simulink model "queuetest_fifth"  (R2018a)
settings: Solver=VariableStepAuto  StartTime=0.0  StopTime=20.0  RelTol=1e-3
undefined symbols (not defined in the file or in its folder): m, n
settings Model: Creator=Michael Girbino  LastModifiedBy=Michael Girbino
settings DebuggingCC: SFNoUnconditionalDefaultTransitionDiag=warning  SFOutputUsedAsStateInMooreChartDiag=warning

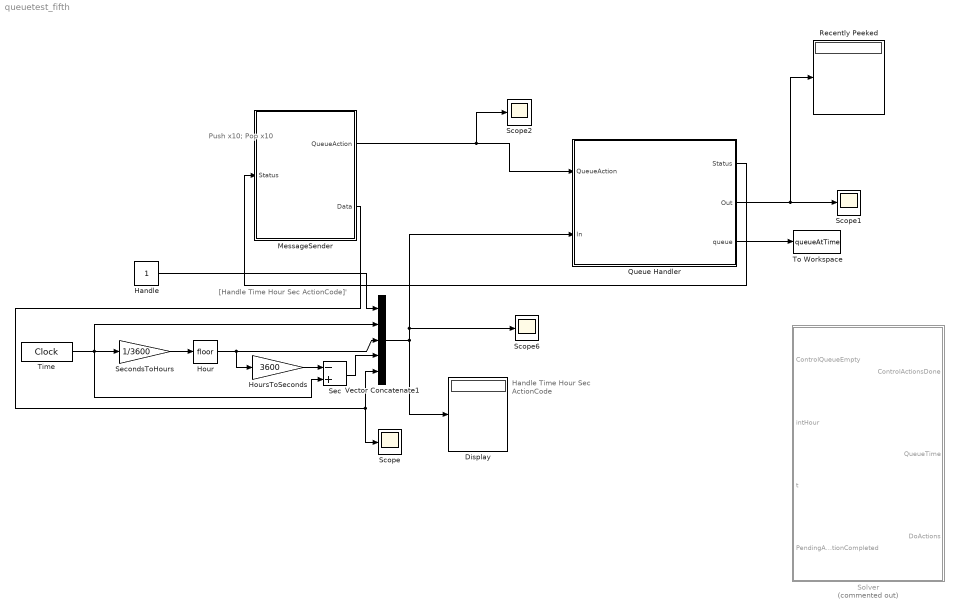
== system queuetest_fifth ==
  note: Push x10;
      | Pop x10
  note: [Handle Time Hour Sec ActionCode]'
  note: Handle
      | Time
      | Hour
      | Sec
      | ActionCode
  Display : Display
  Handle : Constant
  Hour : Rounding
  HoursToSeconds : Gain  Gain=3600
  MessageSender : Stateflow chart  TreatAsAtomicUnit=on
  Queue Handler : Stateflow chart  TreatAsAtomicUnit=on
  Recently Peeked : Display
  Scope{,1..2,6} (4 alike) : Scope
  Sec : Sum  Inputs=-+
  SecondsToHours : Gain  Gain=1/3600
  Solver : Stateflow chart  Commented=on  TreatAsAtomicUnit=on
  Time : DigitalClock
  To Workspace : ToWorkspace  VariableName=queueAtTime  SaveFormat=Structure With Time  SampleTime=-1
  Vector Concatenate1 : Concatenate  NumInputs=5
  wires:
  MessageSender/1(QueueAction) -> Scope2/1, Queue Handler/1(QueueAction)
  MessageSender/2(Data) -> Scope/1, Vector Concatenate1/5
  Queue Handler/1(Status) -> MessageSender/1(Status)
  Queue Handler/2(Out) -> Scope1/1, Recently Peeked/1
  Hour/1 -> Vector Concatenate1/3, HoursToSeconds/1
  Time/1 -> Vector Concatenate1/2, Sec/2, SecondsToHours/1
  SecondsToHours/1 -> Hour/1
  HoursToSeconds/1 -> Sec/1
  Sec/1 -> Vector Concatenate1/4
  Queue Handler/3(queue) -> To Workspace/1
  Handle/1 -> Vector Concatenate1/1
  Vector Concatenate1/1 -> Scope6/1, Queue Handler/2(In), Display/1

== stateflow chart queuetest_fifth/Solver ==
  (default) -> (junction 25) : % Execute control actions in order based on control mode
  (junction 25) -> (junction 26) [order 1] : [ControlMode == ControlModes.STATIC]
  (junction 25) -> (junction 29) [order 2]
  (junction 26) -> (junction 54)
  (junction 54) -> (junction 55) [order 1] : [ControlQueueEmpty]
      | % execute nearest set of control actions, but leave time where it is
  (junction 54) -> (junction 56) [order 2] : {QueueTime = [0,0]; %xHour, xSec
      | DoActions.data = QueueOps.NearestActions;
      | send(DoActions);
      | % ignores time advancement
      | }
  (junction 55) -> (junction 57) : {ControlActionsDone = true;}
  (junction 57) -> (junction 56)
  (junction 56) -> (junction 27)
  (junction 27) -> (junction 28)
  (junction 28) -> (junction 32)
  (junction 29) -> (junction 30) [order 1] : [ControlMode == ControlModes.EVENTDRIVEN]
      | % execute nearest set of control actions and advance time to that time
  (junction 30) -> (junction 65) : {QueueTime = [intHour,t]; %xHour, xSec
      | DoActions.data = QueueOps.NearestActions;
      | send(DoActions);}
  (junction 29) -> (junction 33) [order 2]
  (junction 65) -> (junction 66) [order 1] : [~PendingActionCompleted]
  (junction 65) -> (junction 67) [order 2]
  (junction 66) -> (junction 68) : {ControlActionsDone = true;
      | % advances time to the next event
      | }
  (junction 68) -> (junction 67)
  (junction 67) -> (junction 31)
  (junction 31) -> (junction 32)
  (junction 32) -> (junction 36)
  (junction 33) -> (junction 34) [order 1] : [ControlMode == ControlModes.TIMEDRIVEN]
      |  % Do all actions having and action time <= specified time
  (junction 33) -> (junction 37) [order 2]
  (junction 34) -> (junction 78) : {QueueTime = [intHour,t]; %xHour, xSec
      | DoActions.data = QueueOps.JustActions;
      | send(DoActions);}
  (junction 78) -> (junction 80) [order 1] : [~PendingActionCompleted]
  (junction 78) -> (junction 79) [order 2]
  (junction 80) -> (junction 82) : {ControlActionsDone = true;
      | }
  (junction 82) -> (junction 79)
  (junction 79) -> (junction 35)
  (junction 35) -> (junction 36)
  (junction 36) -> (junction 40)
  (junction 37) -> (junction 38) [order 1] : [ControlMode == ControlModes.MULTIRATE]
      |  % Execute the nearest set of control actions, but leave time where it is
  (junction 37) -> (junction 41) [order 2]
  (junction 38) -> (junction 91) : {QueueTime = [intHour,t]; %xHour, xSec
      | DoActions.data = QueueOps.MultiRate;
      | send(DoActions);}
  (junction 91) -> (junction 88) [order 1] : [~PendingActionCompleted]
  (junction 91) -> (junction 87) [order 2]
  (junction 88) -> (junction 92) : {ControlActionsDone = true;
      | }
  (junction 92) -> (junction 87)
  (junction 87) -> (junction 39)
  (junction 39) -> (junction 40)
  (junction 40) -> (junction 42)
  (junction 42) -> (junction 41)
  (junction 41) -> (junction 43)
  data: ControlQueueEmpty input boolean; ControlActionsDone output boolean; QueueTime output double size=2; DoActions output double; intHour input uint8; t input uint32; PendingActionCompleted input boolean

== stateflow chart queuetest_fifth/MessageSender ==
  settings: enableNonTerminalStates=1
  state SayPush
    en:
    Data = ii;
    QueueAction.data = ...
    QueueActions.PUSH;
    send(QueueAction);
    ii = ii+1;
  state SayPeek
    en:
    QueueAction.data = ...
    QueueActions.PEEK;
    send(QueueAction);
  state SayDoAllACtions
    en:
    QueueAction.data = ...
    QueueActions.DO_ALL_ACTIONS;
    send(QueueAction);
  state SayPop [commented out]
    en:
    QueueAction.data = ...
    QueueActions.POP;
    send(QueueAction);
    ii = ii+1;
  state Asleep
  (default) -> SayPush : {ii = 1;}
  (junction 21) -> SayPush [order 1] : [ii <= 10]
  SayPush -> Asleep [order 2] : Status[Status.data == Statuses.ERROR]
  SayPush -> (junction 21) [order 1] : Status[Status.data == Statuses.READY]
  (junction 21) -> SayPeek [order 2]
  SayPeek -> Asleep [order 2] : Status[Status.data==Statuses.ERROR]
  SayPeek -> (junction 51) [order 1] : Status[Status.data == Statuses.READY]
  (junction 51) -> SayDoAllACtions
  SayDoAllACtions -> Asleep [order 1] : Status[Status.data==Statuses.ERROR]
  SayDoAllACtions -> Asleep [order 2] : {ii = 1;
      | Data = 0;}
  (junction 25) -> SayPop [commented out] : [ii <= 10]
  SayPop -> Asleep [commented out] : Status[Status.data == Statuses.ERROR]
  SayPop -> (junction 25) [commented out] : Status[Status.data == Statuses.READY]
  (junction 25) -> Asleep [commented out]
  data: QueueAction output Enum: QueueActions; Data output double size=1; Status input Enum: Statuses; ii local double =0

== stateflow chart queuetest_fifth/Queue Handler ==
  settings: enableNonTerminalStates=1
  state Executive [parallel]
    settings: executionOrder=1
    state Asleep
      ex: Status.data = Statuses.READY; % reset status
      INTERNAL_DONE = false;
      EXECUTIVE_DONE = false;
    state DoNearestActions
      state WaitOnPeek
        en: send(QUEUE_PEEK, Internal);
      state WaitOnPop
        en: send(QUEUE_POP, Internal);
      state ErrorNoItems
        en: Status.data = ...
        Statuses.ERROR;
        send(Status);
      (default) -> (junction 302) : % do only those actions with the same delay time as the first action time return time
          | {q_len_initial = GetQueueSize;
          | PendingActionsCompleted = false; % local for now
          | }
      (junction 302) -> (junction 315) [order 1] : [q_len_initial > 0]
      (junction 302) -> Executive.DoNearestActions.ErrorNoItems [order 2]
      (junction 315) -> Executive.DoNearestActions.WaitOnPeek : {INTERNAL_DONE = false;}
      (junction 301) -> (junction 331) [order 1] : [jj <= q_len_initial]
      (junction 331) -> Executive.DoNearestActions.WaitOnPop : {INTERNAL_DONE = false;}
      Executive.DoNearestActions.WaitOnPeek -> (junction 301) : [INTERNAL_DONE]
          | {ActionTime = Out(QF.Time);
          | QHour = Out(QF.Hour);
          | QSec = Out(QF.Sec);
          | jj = 1;}
      Executive.DoNearestActions.WaitOnPop -> (junction 299) : [INTERNAL_DONE]
          | %send(DoPendingAction);
      (junction 299) -> (junction 301) : {jj = jj + 1;}
      (junction 301) -> (junction 305) [order 2]
      Executive.DoNearestActions.ErrorNoItems -> (junction 300)
      (junction 305) -> (junction 300)
      (junction 300) -> (junction 298) : {EXECUTIVE_DONE = true;}
    state DoAllActions
      state WaitOnPop
        en: send(QUEUE_POP, Internal);
      state ErrorNoItems
        en: Status.data = ...
        Statuses.ERROR;
        send(Status);
      (default) -> (junction 322) : {q_len_initial = GetQueueSize;}
      (junction 322) -> (junction 321) [order 1] : [q_len_initial ~= 0]
      (junction 322) -> Executive.DoAllActions.ErrorNoItems [order 2]
      (junction 321) -> (junction 326) : {jj = 1;}
      (junction 326) -> (junction 316) [order 1] : [jj <= q_len_initial]
      (junction 316) -> Executive.DoAllActions.WaitOnPop : {INTERNAL_DONE = false;}
      (junction 314) -> (junction 326) : {jj = jj + 1;}
      (junction 326) -> (junction 312) [order 2]
      Executive.DoAllActions.WaitOnPop -> (junction 314) : [INTERNAL_DONE]
          | %send(DoPendingAction);
      Executive.DoAllActions.ErrorNoItems -> (junction 324)
      (junction 312) -> (junction 324)
      (junction 324) -> (junction 310) : {EXECUTIVE_DONE = true;}
    state Pushing
      en: send(QUEUE_PUSH, Internal);
    state Peeking
      en: send(QUEUE_PEEK, Internal);
    state Popping
      en: send(QUEUE_POP, Internal);
    state ReadyAgain
      Status.data = Statuses.READY;
      send(Status);
    Executive.Asleep -> Executive.Peeking [order 5] : QueueAction[QueueAction.data == ...
        | QueueActions.PEEK]
    Executive.Asleep -> Executive.Popping [order 4] : QueueAction[QueueAction.data == ...
        | QueueActions.POP]
    (default) -> Executive.Asleep
    Executive.Asleep -> Executive.Pushing [order 3] : QueueAction[QueueAction.data == ...
        | QueueActions.PUSH]
    Executive.Asleep -> DoAllActions [order 2] : QueueAction[QueueAction.data == ...
        | QueueActions.DO_ALL_ACTIONS]
    ReadyAgain -> Executive.Asleep
    Executive.Asleep -> DoNearestActions [order 1] : QueueAction[QueueAction.data == DO_NEAREST_ACTIONS]
    Executive.Pushing -> ReadyAgain : [INTERNAL_DONE]
    Executive.Popping -> ReadyAgain : [INTERNAL_DONE]
    Executive.Peeking -> ReadyAgain : [INTERNAL_DONE]
    DoAllActions -> ReadyAgain : [EXECUTIVE_DONE]
    DoNearestActions -> ReadyAgain : [EXECUTIVE_DONE]
  state Popping [parallel] [commented out]
    note: FOR TESTING ONLY
    state WaitOnPop [commented out]
    (default) -> Popping.WaitOnPop [commented out] : {send(QUEUE_POP, Internal);}
    Popping.WaitOnPop -> Popping.WaitOnPop [commented out]
    Popping.WaitOnPop -> (junction 625) [commented out] : DONE_POPPING
  state DoNearestActions2 [parallel] [commented out]
    state WaitOnPeek [commented out]
    state PopAction [commented out]
      en: ActionTime = Out(QF.Time);
      QHour = Out(QF.Hour);
      QSec = Out(QF.Sec);
      ii = 1;
      ex: ii = ii +1;
      state WaitOnPop [commented out]
      (default) -> DoNearestActions2.PopAction.WaitOnPop [commented out] : {send(QUEUE_POP);}
      DoNearestActions2.PopAction.WaitOnPop -> DoNearestActions2.PopAction.WaitOnPop [commented out] : [in(Internal.Popping)]
      DoNearestActions2.PopAction.WaitOnPop -> (junction 508) [commented out] : %send(DoPendingAction);
    state ErrorNoItems [commented out]
      en: Status.data = 2;
      send(Status);
    (default) -> (junction 510) [commented out] : % do only those actions with the same delay time as the first action time return time
        | {q_len = size(queue, 3);
        | PendingActionsCompleted = false; % local for now
        | }
    (junction 510) -> (junction 501) [commented out] : [q_len > 0]
    (junction 510) -> DoNearestActions2.ErrorNoItems [commented out]
    (junction 501) -> DoNearestActions2.WaitOnPeek [commented out] : {send(QUEUE_PEEK);}
    DoNearestActions2.WaitOnPeek -> DoNearestActions2.WaitOnPeek [commented out] : [in(Internal.Peeking)]
    DoNearestActions2.WaitOnPeek -> PopAction [commented out]
    PopAction -> PopAction [commented out] : [ii <= q_len]
    DoNearestActions2.ErrorNoItems -> (junction 502) [commented out]
    PopAction -> (junction 498) [commented out]
    (junction 498) -> (junction 502) [commented out]
    (junction 502) -> (junction 499) [commented out]
  state Peeking [parallel] [commented out]
    note: FOR TESTING ONLY
    state WaitOnPeek [commented out]
    (default) -> Peeking.WaitOnPeek [commented out] : {send(QUEUE_PEEK, Internal);}
    Peeking.WaitOnPeek -> Peeking.WaitOnPeek [commented out] : [in(Internal.Peeking)]
    Peeking.WaitOnPeek -> (junction 619) [commented out]
  state Pushing1 [parallel] [commented out]
    state WaitOnPush [commented out]
    (default) -> WaitOnPush [commented out] : {send(QUEUE_PUSH, Internal);}
    WaitOnPush -> (junction 610) [commented out] : [INTERNAL_DONE]
        | {EXECUTIVE_DONE = true;}
  state Internal [parallel]
    settings: executionOrder=2
    state Asleep
    state Popping
      (default) -> (junction 163) : % delete from beginning, t<= ActionTime:
          | {q_len = GetQueueSize;
          | ii = 1;
          | }
      (junction 163) -> (junction 169) [order 1] : [ii <= q_len]
      (junction 169) -> (junction 157)
      (junction 157) -> (junction 158) [order 1] : [GetElemTime(ii) <= ActionTime]
      (junction 157) -> (junction 164) [order 2]
      (junction 158) -> (junction 159) : {Out = GetElem(ii);
          | ReduceQueue(ii);}
          | % break
      (junction 164) -> (junction 163) : {ii = ii + 1;}
      (junction 163) -> (junction 165) [order 2]
      (junction 159) -> (junction 165)
      (junction 165) -> (junction 162) : %{send(DONE_POPPING, Executive.Popping);}
          | {INTERNAL_DONE = true;}
    state Pushing
      (default) -> (junction 136) : % insert into queue right before item of greater or equal execution time
          | {q_cand = In'; % transposition to 1 x 5
          | q_len = GetQueueSize; %size(queue, 3);
          | ii = 1;
          | }
      (junction 136) -> (junction 134) [order 1] : [ii <= q_len]
      (junction 134) -> (junction 145)
      (junction 145) -> (junction 146) [order 1] : [q_cand(1,QF.Time) <= GetElemTime(ii)]
      (junction 145) -> (junction 137) [order 2]
      (junction 146) -> (junction 148) : {
          | ExpandQueue(ii);}
          | % break
      (junction 137) -> (junction 136) : {ii = ii + 1;}
      (junction 136) -> (junction 138) [order 2] : {ExpandQueue(q_len+1);}
      (junction 148) -> (junction 138)
      (junction 138) -> (junction 151) : %{send(DONE_PUSHING, Executive.Pushing);}
          | {INTERNAL_DONE = true;}
    state Peeking
      (default) -> (junction 181) : % pop without deletion
          | {q_len = GetQueueSize;
          | ii = 1;
          | }
      (junction 181) -> (junction 187) [order 1] : [ii <= q_len]
      (junction 187) -> (junction 175)
      (junction 175) -> (junction 176) [order 1] : [GetElemTime(ii) <= ActionTime]
      (junction 175) -> (junction 182) [order 2]
      (junction 176) -> (junction 177) : {Out = GetElem(ii);}
          | % break
      (junction 182) -> (junction 181) : {ii = ii + 1;}
      (junction 181) -> (junction 183) [order 2]
      (junction 177) -> (junction 183)
      (junction 183) -> (junction 180) : {INTERNAL_DONE = true;}
    (default) -> Internal.Asleep
    Internal.Asleep -> Internal.Pushing [order 1] : QUEUE_PUSH
    Internal.Pushing -> Internal.Asleep : [INTERNAL_DONE]
    Internal.Asleep -> Internal.Popping [order 2] : QUEUE_POP
    Internal.Popping -> Internal.Asleep : [INTERNAL_DONE]
    Internal.Asleep -> Internal.Peeking [order 3] : QUEUE_PEEK
    Internal.Peeking -> Internal.Asleep : [INTERNAL_DONE]
  state QF % Queue Fields [group]
  data: Handle local double =1; Time local double =2; Hour local double =3; Sec local double =4; ActionCode local double =5; qs function_output; depth function_input; et function_output; elem function_output; depth function_input; depth function_input; depth function_input; QueueAction input Enum: QueueActions; Status output Enum: Statuses; Out output double size=[1 5]; queue output double size=[1 5 50]; q_len local double =0; ActionTime local double =100; PendingActionsCompleted local boolean =false; QHour local double; QSec local double; q_cand local double size=[1 5]; In input double size=5; qwriteflag local boolean =false; ii local uint8; jj local uint8; q_len_initial local double; DONE_PUSHING local; EXECUTIVE_DONE local boolean =false; INTERNAL_DONE local boolean =false;
  events: QUEUE_POP local FUNCTION_CALL_EVENT; QUEUE_PUSH local FUNCTION_CALL_EVENT; QUEUE_PEEK local FUNCTION_CALL_EVENT; DONE_POPPING local FUNCTION_CALL_EVENT
  function qs = GetQueueSize:
    | function qs = GetQueueSize
    | %     coder.extrinsic('exist');
    | %     eq = zeros(1,1,'double');
    | %     eq = exist('queue');
    | %     if eq == 1 && ~isempty(queue)
    | %         qs = size(queue, 3);
    | %     else % eq ~= 1 || size == 0
    | %         qs = 0;
    | %     end
    |     if ~qwriteflag % can't read intial value of empty queue, so depend on flag
    |         queue = zeros(1,5);
    |         qs = 0;
    |         qwriteflag = true;
    |     elseif isequal(queue,zeros(1,5)) % case of empty queue (still 1 element)
    |         qs = 0;
    |     else
    |         qs = size(queue,3);
    |     end
    | end
  function et = GetElemTime(depth):
    | function et = GetElemTime(depth)
    |     et = zeros(1,1);
    |     if ~isempty(queue)
    |         et = queue(1,QF.Time,ii);
    |     else
    |     end
    | end
  function elem = GetElem(depth):
    | function elem = GetElem(depth)
    |     elem = zeros(1,5);
    |     elem(1,:) = queue(:,:,depth);
    | end
  function ExpandQueue(depth):
    | function ExpandQueue(depth)
    |     rhs = queue(:,:,depth:q_len); % the RHS of the queue
    |     bigger = zeros(1,5,q_len+1);
    |     bigger(:,:,1:(depth-1)) = queue(:,:,1:(depth-1)); % copy LHS
    |     bigger(:,:,depth) = q_cand; % inserting element at end of LHS
    |     %queue(:,:,depth) = q_cand; 
    |     bigger(:,:, (depth+1):(q_len+1)) = rhs; % tack on RHS again
    |     queue = bigger;
    | end
  function ReduceQueue(depth):
    | function ReduceQueue(depth)
    |     rhs = queue(:,:,(depth+1):q_len); % excluding element at depth
    |     smaller = zeros(1,5,q_len-1);
    |     smaller(:,:,1:(depth-1)) = queue(:,:,1:(depth-1)); % lhs, excl. depth
    |     smaller(:,:,depth:(q_len-1)) = rhs; % tack on rhs
    |     queue = smaller;
    | end
